simulink model "testHarness9CombinedFreqBlocks"  (R2018b)
settings: Solver=ode23s  StartTime=0.0  StopTime=7000  MaxStep=0.1*sqrt(sim.lengthScaleFactor.Value)  RelTol=1e-3  AbsTol=1e-3
libraries: combinedHighLowFreqData_cl x9
settings Model: SimulationMode=accelerator  Creator=jcreed2  LastModifiedBy=jcreed2

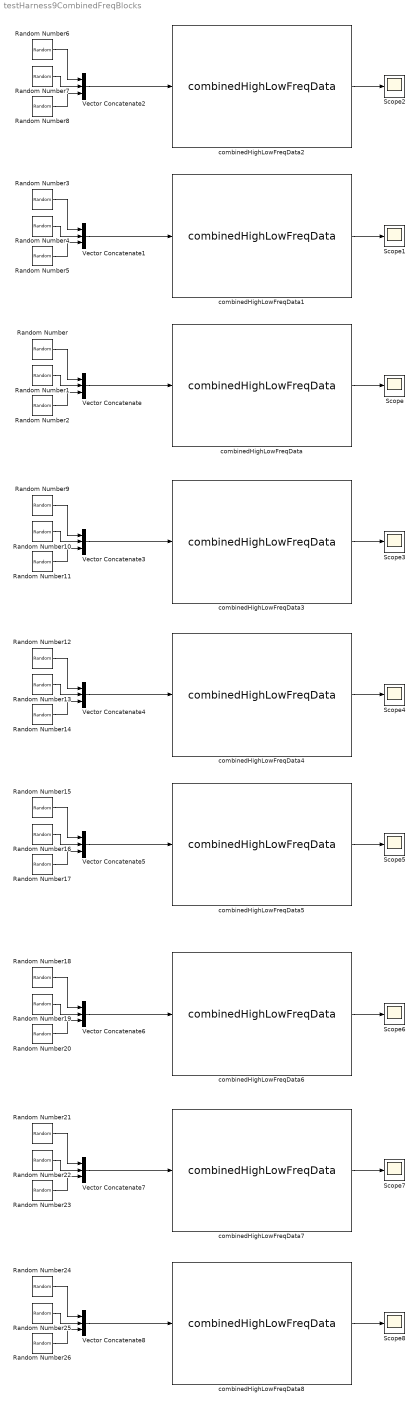
== system testHarness9CombinedFreqBlocks ==
  Random Number{,1..26} (27 alike) : RandomNumber  SampleTime=0.1
  Scope{,1..8} (9 alike) : Scope
  Vector Concatenate{,1..8} (9 alike) : Concatenate  NumInputs=3
  combinedHighLowFreqData{,1..8} (9 alike) : combinedHighLowFreqData_cl/combinedHighLowFreqData  VariantControl=VSS_flowCalculation_combinedHighLowFreqData  flw=env.water  hFlw=env.waterTurb
  wires:
  combinedHighLowFreqData/1 -> Scope/1
  Vector Concatenate/1 -> combinedHighLowFreqData/1
  Random Number/1 -> Vector Concatenate/1
  Random Number1/1 -> Vector Concatenate/2
  Random Number2/1 -> Vector Concatenate/3
  Vector Concatenate1/1 -> combinedHighLowFreqData1/1
  Random Number5/1 -> Vector Concatenate1/3
  Random Number3/1 -> Vector Concatenate1/1
  Random Number4/1 -> Vector Concatenate1/2
  combinedHighLowFreqData1/1 -> Scope1/1
  Vector Concatenate2/1 -> combinedHighLowFreqData2/1
  Random Number8/1 -> Vector Concatenate2/3
  Random Number6/1 -> Vector Concatenate2/1
  Random Number7/1 -> Vector Concatenate2/2
  combinedHighLowFreqData2/1 -> Scope2/1
  Vector Concatenate3/1 -> combinedHighLowFreqData3/1
  Random Number11/1 -> Vector Concatenate3/3
  Random Number9/1 -> Vector Concatenate3/1
  Random Number10/1 -> Vector Concatenate3/2
  combinedHighLowFreqData3/1 -> Scope3/1
  Vector Concatenate4/1 -> combinedHighLowFreqData4/1
  Random Number14/1 -> Vector Concatenate4/3
  Random Number12/1 -> Vector Concatenate4/1
  Random Number13/1 -> Vector Concatenate4/2
  combinedHighLowFreqData4/1 -> Scope4/1
  Vector Concatenate5/1 -> combinedHighLowFreqData5/1
  Random Number17/1 -> Vector Concatenate5/3
  Random Number15/1 -> Vector Concatenate5/1
  Random Number16/1 -> Vector Concatenate5/2
  combinedHighLowFreqData5/1 -> Scope5/1
  Vector Concatenate6/1 -> combinedHighLowFreqData6/1
  Random Number20/1 -> Vector Concatenate6/3
  Random Number18/1 -> Vector Concatenate6/1
  Random Number19/1 -> Vector Concatenate6/2
  combinedHighLowFreqData6/1 -> Scope6/1
  Vector Concatenate7/1 -> combinedHighLowFreqData7/1
  combinedHighLowFreqData7/1 -> Scope7/1
  Random Number23/1 -> Vector Concatenate7/3
  Random Number22/1 -> Vector Concatenate7/2
  Random Number21/1 -> Vector Concatenate7/1
  Vector Concatenate8/1 -> combinedHighLowFreqData8/1
  combinedHighLowFreqData8/1 -> Scope8/1
  Random Number26/1 -> Vector Concatenate8/3
  Random Number25/1 -> Vector Concatenate8/2
  Random Number24/1 -> Vector Concatenate8/1
